simulink model "LQR_model"  (R2020a)
settings: Solver=VariableStepAuto  StartTime=0.0  StopTime=10  RelTol=1e-3
values from neighbouring files (symbols this model uses):
  A = [0 0 0 1 0 0 0 0 0 0 0 0 ... (first row only)    [quadrotor_parameters.m]
  B = [0 0 0 0 ... (first row only)    [quadrotor_parameters.m]
  C = [0 0 1 0 0 0 0 0 0 0 0 0 ... (first row only)    [quadrotor_parameters.m]
  G = L*J    [quadrotor_parameters.m]
  kf = 9.8e-6    (= 9.8e-06)    [quadrotor_parameters.m]
  km = 1.6e-7    (= 1.6e-07)    [quadrotor_parameters.m]
  w1 = 100    [quadrotor_parameters.m]
  w2 = 100    [quadrotor_parameters.m]
  w3 = 100    [quadrotor_parameters.m]
  w4 = 100    [quadrotor_parameters.m]
undefined symbols (not defined in the file or in its folder): K
settings Model: Creator=Dr.Saraf  LastModifiedBy=Dr.Saraf
settings DataIOCC: ReturnWorkspaceOutputs=off
settings DebuggingCC: ArithmeticOperatorsInVariantConditions=warning
settings SFSimCC: SimUseLocalCustomCode=off  CustomCodeUndefinedFunction=UseInterfaceOnly
settings RTWCC: RTWUseLocalCustomCode=off
settings CodeAppCC: StateflowObjectComments=on

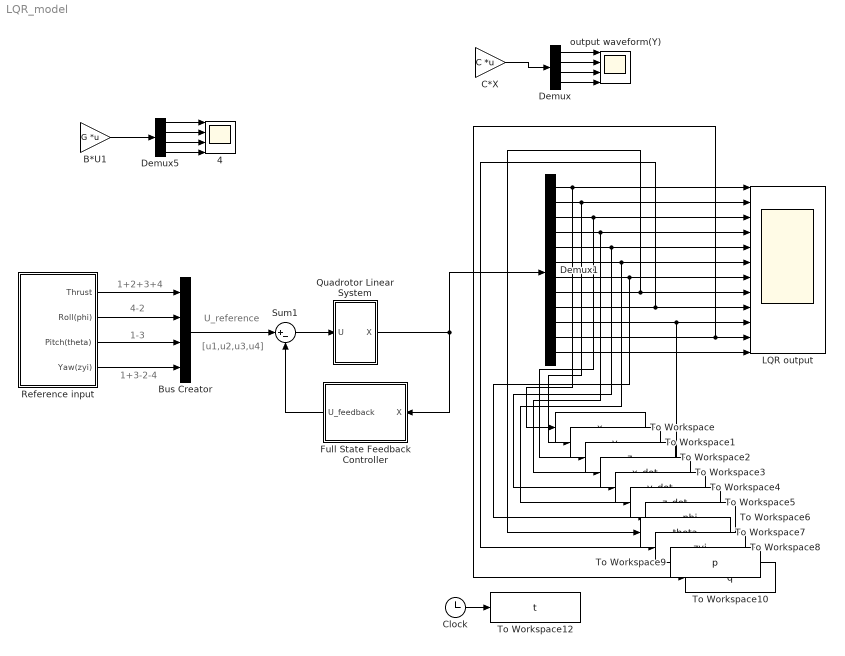
== system LQR_model ==
  note: U_reference
  note: 1+2+3+4
  note: 1+3-2-4
  note: 1-3
  note: 4-2
  note: [u1,u2,u3,u4]
  4 : Scope  NumInputPorts=4
  B*U1 : Gain  Gain=G  Multiplication=Matrix(K*u)
  Bus Creator : BusCreator  Inputs=4
  C*X : Gain  Gain=C  Multiplication=Matrix(K*u)
  Clock : Clock
  Demux : Demux
  Demux1 : Demux  Outputs=12
  Demux5 : Demux
  Full State Feedback Controller : Subsystem
  "LQR output " : Scope  NumInputPorts=12
  Quadrotor Linear System : Subsystem
  Reference input : Subsystem
  Sum1 : Sum  Inputs=|+-
  To Workspace : ToWorkspace  VariableName=x  SampleTime=0.1
  To Workspace1 : ToWorkspace  VariableName=y  SampleTime=0.1
  To Workspace10 : ToWorkspace  VariableName=q  SampleTime=0.1
  To Workspace12 : ToWorkspace  VariableName=t  SampleTime=0.001
  To Workspace2 : ToWorkspace  VariableName=z  SampleTime=0.1
  To Workspace3 : ToWorkspace  VariableName=x_dot  SampleTime=0.1
  To Workspace4 : ToWorkspace  VariableName=y_dot  SampleTime=0.1
  To Workspace5 : ToWorkspace  VariableName=z_dot  SampleTime=0.1
  To Workspace6 : ToWorkspace  VariableName=phi  SampleTime=0.1
  To Workspace7 : ToWorkspace  VariableName=theta  SampleTime=0.1
  To Workspace8 : ToWorkspace  VariableName=zyi  SampleTime=0.1
  To Workspace9 : ToWorkspace  VariableName=p  SampleTime=0.1
  output waveform(Y) : Scope  NumInputPorts=4
  wires:
  Demux1/2 -> To Workspace1/1, "LQR output "/2
  Demux1/3 -> To Workspace2/1, "LQR output "/3
  Demux/3 -> output waveform(Y)/3
  Demux1/4 -> To Workspace3/1, "LQR output "/4
  Demux/1 -> output waveform(Y)/1
  Bus Creator/1 -> Sum1/1
  Demux1/9 -> To Workspace8/1, "LQR output "/9
  Demux1/12 -> "LQR output "/12
  Demux/4 -> output waveform(Y)/4
  Demux/2 -> output waveform(Y)/2
  Demux1/7 -> To Workspace6/1, "LQR output "/7
  Demux1/11 -> To Workspace10/1, "LQR output "/11
  Demux1/6 -> To Workspace5/1, "LQR output "/6
  Demux1/5 -> To Workspace4/1, "LQR output "/5
  Demux1/10 -> To Workspace9/1, "LQR output "/10
  Demux1/8 -> To Workspace7/1, "LQR output "/8
  Demux1/1 -> To Workspace/1, "LQR output "/1
  C*X/1 -> Demux/1
  Reference input/1(Thrust) -> Bus Creator/1
  Reference input/2(Roll(phi)) -> Bus Creator/2
  Reference input/3(Pitch(theta)) -> Bus Creator/3
  Reference input/4(Yaw(zyi)) -> Bus Creator/4
  Demux5/1 -> 4/1
  Demux5/2 -> 4/2
  Demux5/4 -> 4/4
  Demux5/3 -> 4/3
  B*U1/1 -> Demux5/1
  Sum1/1 -> Quadrotor Linear System/1(U)
  Quadrotor Linear System/1(X) -> Demux1/1, Full State Feedback Controller/1(X)
  Full State Feedback Controller/1(U_feedback) -> Sum1/2
  Clock/1 -> To Workspace12/1

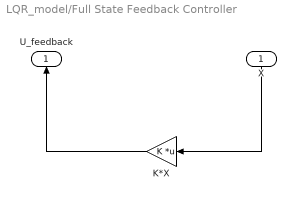
== system LQR_model/Full State Feedback Controller ==
  X : Inport
  K*X : Gain  Gain=K  Multiplication=Matrix(K*u)
  U_feedback : Outport
  wires:
  K*X/1 -> U_feedback/1
  X/1 -> K*X/1

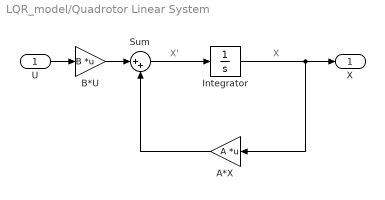
== system LQR_model/Quadrotor Linear System ==
  note: X'
  note: X
  U : Inport
  A*X : Gain  Gain=A  Multiplication=Matrix(K*u)
  B*U : Gain  Gain=B  Multiplication=Matrix(K*u)
  Integrator : Integrator  InitialCondition=[1,1,1,1,1,1,1,1,1,1,1,1]
  Sum : Sum  Inputs=|++
  X : Outport
  wires:
  U/1 -> B*U/1
  A*X/1 -> Sum/2
  Sum/1 -> Integrator/1
  B*U/1 -> Sum/1
  Integrator/1 -> X/1, A*X/1

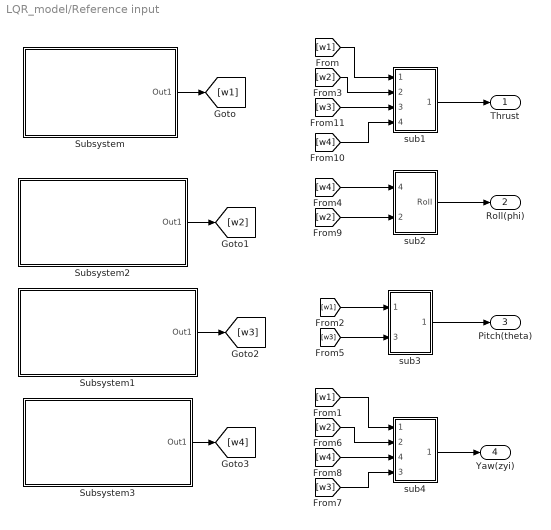
== system LQR_model/Reference input ==
  Subsystem : Subsystem
  Subsystem1 : Subsystem
  Subsystem2 : Subsystem
  Subsystem3 : Subsystem
  sub1 : Subsystem
  "sub2 " : Subsystem
  "sub3 " : Subsystem
  sub4 : Subsystem
  Thrust : Outport
  Roll(phi) : Outport  Port=2
  Pitch(theta) : Outport  Port=3
  Yaw(zyi) : Outport  Port=4
  wires:
  [w4] -> sub1/4(4)
  [w3] -> sub1/3(3)
  [w2] -> sub1/2(2)
  [w1] -> sub4/1(1)
  [w4] -> sub4/3("4 ")
  [w3] -> sub4/4("3 ")
  [w1] -> "sub3 "/1(1)
  [w4] -> "sub2 "/1(4)
  [w3] -> "sub3 "/2(3)
  [w1] -> sub1/1(1)
  [w2] -> sub4/2(2)
  [w2] -> "sub2 "/2(2)
  "sub2 "/1(Roll) -> Roll(phi)/1
  sub1/1(Thrust) -> Thrust/1
  sub4/1(Yaw) -> Yaw(zyi)/1
  "sub3 "/1(Pitch) -> Pitch(theta)/1
  Subsystem1/1(Out1) -> [w3]
  Subsystem/1(Out1) -> [w1]
  Subsystem2/1(Out1) -> [w2]
  Subsystem3/1(Out1) -> [w4]

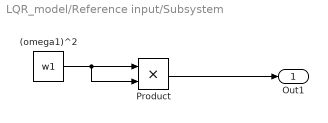
== system LQR_model/Reference input/Subsystem ==
  (omega1)^2 : Constant  Value=w1
  Product : Product
  Out1 : Outport
  wires:
  (omega1)^2/1 -> Product/2, Product/1
  Product/1 -> Out1/1

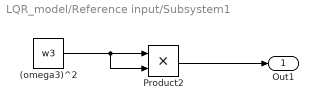
== system LQR_model/Reference input/Subsystem1 ==
  (omega3)^2 : Constant  Value=w3
  Product2 : Product
  Out1 : Outport
  wires:
  (omega3)^2/1 -> Product2/2, Product2/1
  Product2/1 -> Out1/1

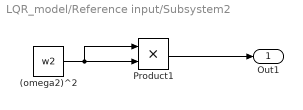
== system LQR_model/Reference input/Subsystem2 ==
  (omega2)^2 : Constant  Value=w2
  Product1 : Product
  Out1 : Outport
  wires:
  (omega2)^2/1 -> Product1/1, Product1/2
  Product1/1 -> Out1/1

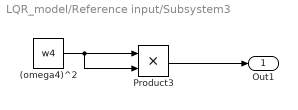
== system LQR_model/Reference input/Subsystem3 ==
  (omega4)^2 : Constant  Value=w4
  Product3 : Product
  Out1 : Outport
  wires:
  (omega4)^2/1 -> Product3/2, Product3/1
  Product3/1 -> Out1/1

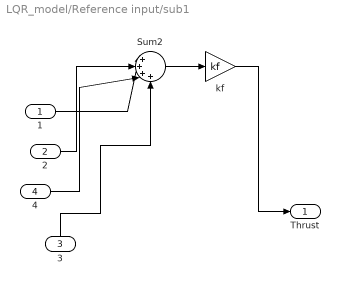
== system LQR_model/Reference input/sub1 ==
  1 : Inport
  2 : Inport  Port=2
  3 : Inport  Port=3
  4 : Inport  Port=4
  Sum2 : Sum  Inputs=|++++
  kf : Gain  Gain=kf
  Thrust : Outport
  wires:
  kf/1 -> Thrust/1
  Sum2/1 -> kf/1
  1/1 -> Sum2/1
  2/1 -> Sum2/2
  3/1 -> Sum2/4
  4/1 -> Sum2/3

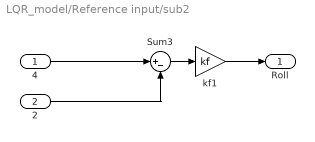
== system LQR_model/Reference input/sub2  ==
  4 : Inport
  2 : Inport  Port=2
  Sum3 : Sum  Inputs=|+-
  kf1 : Gain  Gain=kf
  Roll : Outport
  wires:
  kf1/1 -> Roll/1
  Sum3/1 -> kf1/1
  4/1 -> Sum3/1
  2/1 -> Sum3/2

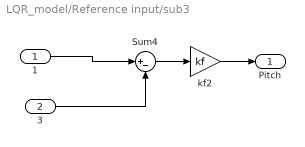
== system LQR_model/Reference input/sub3  ==
  1 : Inport
  3 : Inport  Port=2
  Sum4 : Sum  Inputs=|+-
  kf2 : Gain  Gain=kf
  Pitch : Outport
  wires:
  3/1 -> Sum4/2
  1/1 -> Sum4/1
  Sum4/1 -> kf2/1
  kf2/1 -> Pitch/1

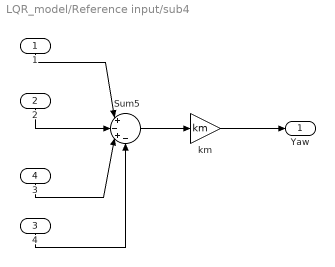
== system LQR_model/Reference input/sub4 ==
  1 : Inport
  2 : Inport  Port=2
  "4 " : Inport  Port=3
  "3 " : Inport  Port=4
  Sum5 : Sum  Inputs=|+-+-
  km : Gain  Gain=km
  Yaw : Outport
  wires:
  Sum5/1 -> km/1
  km/1 -> Yaw/1
  "3 "/1 -> Sum5/3
  2/1 -> Sum5/2
  "4 "/1 -> Sum5/4
  1/1 -> Sum5/1
